simulink model "lab02es1"  (R2021b)
settings: Solver=VariableStepAuto  StartTime=0.0  StopTime=10  RelTol=1e-3
undefined symbols (not defined in the file): m, n
settings Model: Creator=francescafornasier  LastModifiedBy=francescafornasier

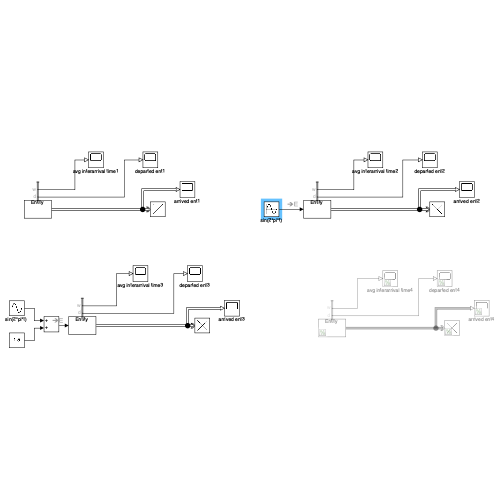
[thumbnail: Simulink's stored preview of the top-level diagram]
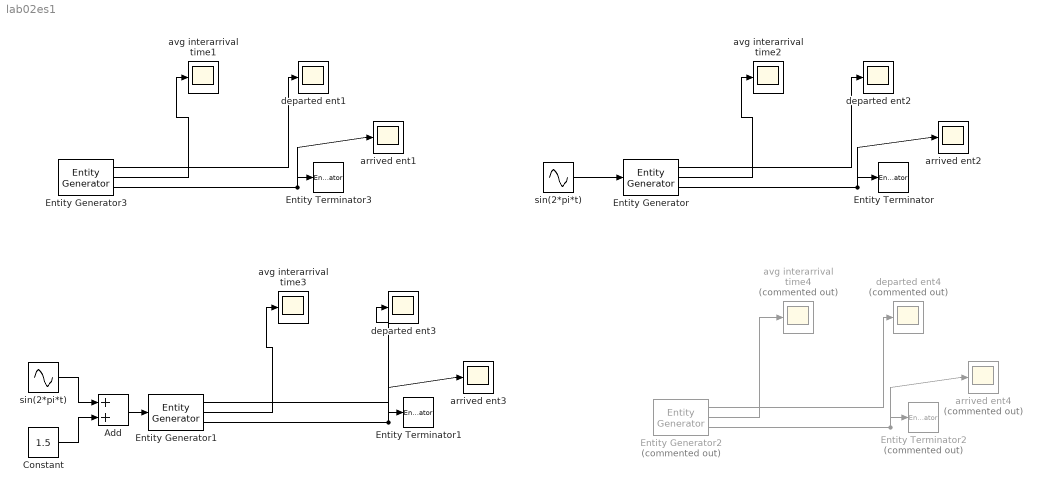
== system lab02es1 ==
  Add : Sum
  Constant : Constant  Value=1.5
  Entity Generator : EntityGenerator  OutputPortMessageModes=n,n,m  TimeSource=Signal port  Period=0.5  IntergenerationTimeAction=dt = exprnd(0.5);  NumberEntitiesDeparted=on  AverageIntergenerationTime=on  EntityType=Structured  EntityTypeName=Entity
      settings: InputPortMap=u1  OutputPortMap=o0,o2,o3
  Entity Generator1 : EntityGenerator  OutputPortMessageModes=n,n,m  TimeSource=Signal port  Period=0.5  IntergenerationTimeAction=dt = exprnd(0.5);  GenerateEntityAtSimulationStart=off  NumberEntitiesDeparted=on  AverageIntergenerationTime=on  EntityType=Structured  EntityTypeName=Entity
      settings: InputPortMap=u1  OutputPortMap=o0,o2,o3
  Entity Generator2 : EntityGenerator  Commented=on  OutputPortMessageModes=n,n,m  TimeSource=MATLAB action  Period=0.5  IntergenerationTimeAction=dt = exprnd(0.5);  NumberEntitiesDeparted=on  AverageIntergenerationTime=on  EntityType=Structured  EntityTypeName=Entity
      settings: OutputPortMap=o0,o2,o3
  Entity Generator3 : EntityGenerator  OutputPortMessageModes=n,n,m  Period=0.5  IntergenerationTimeAction=dt = exprnd(0.5);  NumberEntitiesDeparted=on  AverageIntergenerationTime=on  EntityType=Structured  EntityTypeName=Entity
      settings: OutputPortMap=o0,o2,o3
  Entity Terminator : EntityTerminator  InputPortMessageModes=m
  Entity Terminator1 : EntityTerminator  InputPortMessageModes=m
  Entity Terminator2 : EntityTerminator  Commented=on  InputPortMessageModes=m
  Entity Terminator3 : EntityTerminator  InputPortMessageModes=m
  arrived ent1 : Scope
  arrived ent2 : Scope
  arrived ent3 : Scope
  arrived ent4 : Scope  Commented=on
  avg interarrival time1 : Scope
  avg interarrival time2 : Scope
  avg interarrival time3 : Scope
  avg interarrival time4 : Scope  Commented=on
  departed ent1 : Scope
  departed ent2 : Scope
  departed ent3 : Scope
  departed ent4 : Scope  Commented=on
  sin(2*pi*t) : Sin  Frequency=2*pi  Phase=pi/2  SampleTime=0
  "sin(2*pi*t) " : Sin  Frequency=2*pi  SampleTime=0
  wires:
  Entity Generator/2 -> avg interarrival time2/1
  Entity Generator/1 -> departed ent2/1
  Entity Generator/3 -> arrived ent2/1, Entity Terminator/1
  Entity Generator1/3 -> arrived ent3/1, Entity Terminator1/1
  Entity Generator1/2 -> avg interarrival time3/1
  Entity Generator1/1 -> departed ent3/1
  Entity Generator2/2 -> avg interarrival time4/1
  Entity Generator2/3 -> arrived ent4/1, Entity Terminator2/1
  Entity Generator2/1 -> departed ent4/1
  sin(2*pi*t)/1 -> Entity Generator/1
  Add/1 -> Entity Generator1/1
  Constant/1 -> Add/2
  "sin(2*pi*t) "/1 -> Add/1
  Entity Generator3/1 -> departed ent1/1
  Entity Generator3/2 -> avg interarrival time1/1
  Entity Generator3/3 -> arrived ent1/1, Entity Terminator3/1
